simulink model "Copy_of_PF_implementacion_modeloNL2"  (R2023a)
settings: Solver=ode15s  StartTime=0.0  StopTime=t_sim  RelTol=1e-3
values from neighbouring files (symbols this model uses):
  F_in_fin = F_in    (= 2)    [PF_CP_Completo_Level2.m]
  F_in_ini = F_in    (= 2)    [PF_CP_Completo_Level2.m]
  L_in_fin = L_in*1.5    (= 0)    [PF_CP_Completo_Level2.m]
  L_in_ini = L_in    (= 0)    [PF_CP_Completo_Level2.m]
  ODE_ss = [y_out(end,1),y_out(end,2),y_out(end,3),y_out(end,4),y_out(end,5)]    [PF_CP_Completo_Level2.m]
  Q_in_fin = Q_in    (= 0)    [PF_CP_Completo_Level2.m]
  Q_in_ini = Q_in    (= 0)    [PF_CP_Completo_Level2.m]
  S1_in_fin = S1_in    (= 60)    [PF_CP_Completo_Level2.m]
  S1_in_ini = S1_in    (= 60)    [PF_CP_Completo_Level2.m]
  S2_in_fin = S2_in    (= 20)    [PF_CP_Completo_Level2.m]
  S2_in_ini = S2_in    (= 20)    [PF_CP_Completo_Level2.m]
  t_step = 200    [PF_CP_Completo_Level2.m]
  x_in_fin = x_in    (= 0)    [PF_CP_Completo_Level2.m]
  x_in_ini = x_in    (= 0)    [PF_CP_Completo_Level2.m]
undefined symbols (not defined in the file or in its folder): A1, B1, C1, D1
settings Model: Creator=ja616  LastModifiedBy=ja616

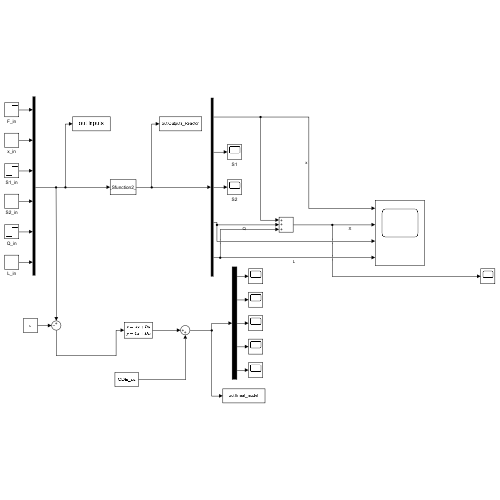
[thumbnail: Simulink's stored preview of the top-level diagram]
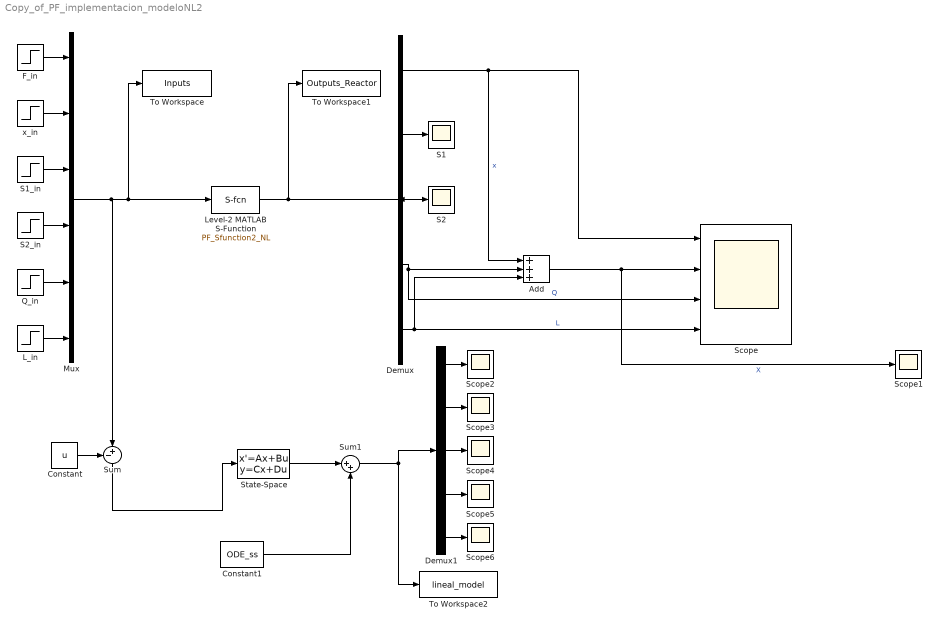
== system Copy_of_PF_implementacion_modeloNL2 ==
  Add : Sum  Inputs=+++
  Constant : Constant  Value=u
  Constant1 : Constant  Value=ODE_ss
  Demux : Demux  Outputs=5
  Demux1 : Demux  Outputs=5
  F_in : Step  Time=t_step  Before=F_in_ini  After=F_in_fin  SampleTime=0
  L_in : Step  Time=t_step  Before=L_in_ini  After=L_in_fin  SampleTime=0
  Level-2 MATLAB S-Function : M-S-Function  FunctionName=PF_Sfunction2_NL
  Mux : Mux  Inputs=6
  Q_in : Step  Time=t_step  Before=Q_in_ini  After=Q_in_fin  SampleTime=0
  S1 : Scope
  S1_in : Step  Time=t_step  Before=S1_in_ini  After=S1_in_fin  SampleTime=0
  S2 : Scope
  S2_in : Step  Time=t_step  Before=S2_in_ini  After=S2_in_fin  SampleTime=0
  Scope : Scope  NumInputPorts=4
  Scope{1..6} (6 alike) : Scope
  State-Space : StateSpace  A=A1  B=B1  C=C1  D=D1  InitialCondition=0
  Sum : Sum  Inputs=-+|
  Sum1 : Sum  Inputs=|++
  To Workspace : ToWorkspace  VariableName=Inputs  SaveFormat=Timeseries  SampleTime=-1
  To Workspace1 : ToWorkspace  VariableName=Outputs_Reactor  SaveFormat=Timeseries  SampleTime=-1
  To Workspace2 : ToWorkspace  VariableName=lineal_model  SaveFormat=Timeseries  SampleTime=-1
  x_in : Step  Time=t_step  Before=x_in_ini  After=x_in_fin  SampleTime=0
  wires:
  F_in/1 -> Mux/1
  Mux/1 -> Sum/2, Level-2 MATLAB S-Function/1, To Workspace/1
  L_in/1 -> Mux/6
  S2_in/1 -> Mux/4
  S1_in/1 -> Mux/3
  Level-2 MATLAB S-Function/1 -> Demux/1, To Workspace1/1
  Q_in/1 -> Mux/5
  x_in/1 -> Mux/2
  Demux/1 -> Scope/1, Add/1  "x"
  Demux/2 -> S1/1
  Demux/3 -> S2/1
  Demux/4 -> Scope/3, Add/2  "Q"
  Demux/5 -> Add/3, Scope/4  "L"
  Add/1 -> Scope1/1, Scope/2  "X"
  Constant/1 -> Sum/1
  Sum/1 -> State-Space/1
  State-Space/1 -> Sum1/1
  Sum1/1 -> To Workspace2/1, Demux1/1
  Demux1/1 -> Scope2/1
  Demux1/2 -> Scope3/1
  Demux1/3 -> Scope4/1
  Demux1/4 -> Scope5/1
  Demux1/5 -> Scope6/1
  Constant1/1 -> Sum1/2
